simulink model "stateFullOBS"  (Simulink 7.4)
settings: Solver=ode4  StartTime=0.0  StopTime=inf  FixedStep=0.01  RelTol=1e-3
undefined symbols (not defined in the file): A, aarm, apind, B, C, F, Fi, L, M
libraries: xpcnilib x2
settings Model: Creator=Skov  LastModifiedBy=Skov  SimulationMode=external  BufferReuse=off
settings DataIOCC: SaveState=on  InspectSignalLogs=on
settings OptimizationCC: BlockReduction=off  OptimizeBlockIOStorage=off  BufferReuse=off  ExpressionFolding=off  LocalBlockOutputs=off
settings HardwareCC: ProdIntDivRoundTo=Zero  ProdEndianess=LittleEndian  ProdHWDeviceType=Generic->32-bit x86 compatible
settings RTWCC: SystemTargetFile=xpctarget.tlc  TemplateMakefile=xpc_default_tmf  Description=xPC Target  ProcessScript=xpctarget_make_rtw_hook  RTWCompilerOptimization=On
settings xpcTargetCC: TargetFcnLib=ansi_tfl_table_tmw.mat  TargetFunctionLibrary=ANSI_C  ParMdlRefBuildCompliant=off  PortableWordSizes=off  xPCLoadParamSetFile=off

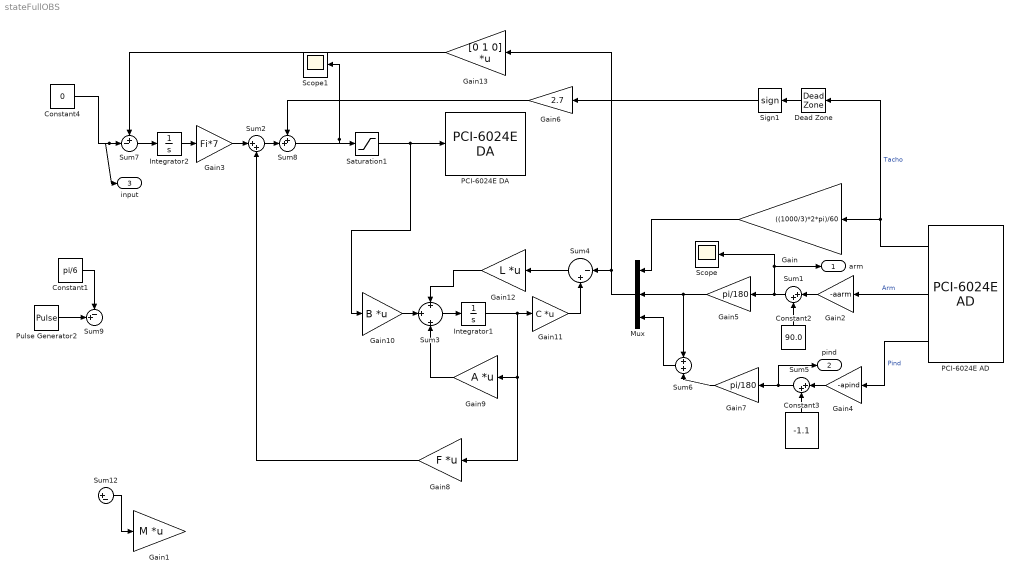
== system stateFullOBS ==
  Constant1 : Constant  Value=pi/6  OutDataType=fixdt(1, 16)  OutScaling=2^0
  Constant2 : Constant  Value=90.0  OutDataType=fixdt(1, 16)  OutScaling=2^0
  Constant3 : Constant  Value=-1.1  OutDataType=fixdt(1, 16)  OutScaling=2^0
  Constant4 : Constant  Value=0  OutDataType=fixdt(1, 16)  OutScaling=2^0
  Dead Zone : DeadZone  LowerValue=-0.01  UpperValue=0.01  SaturateOnIntegerOverflow=on
  Gain : Gain  Gain=((1000/3)*2*pi)/60  ParameterDataType=fixdt(1, 16)  ParameterScaling=2^0  OutDataType=fixdt(1, 16)  OutScaling=2^0
  Gain1 : Gain  Gain=M  Multiplication=Matrix(K*u)  ParameterDataType=fixdt(1, 16)  ParameterScaling=2^0  OutDataType=fixdt(1, 16)  OutScaling=2^0
  Gain10 : Gain  Gain=B  Multiplication=Matrix(K*u)  ParameterDataType=fixdt(1, 16)  ParameterScaling=2^0  OutDataType=fixdt(1, 16)  OutScaling=2^0
  Gain11 : Gain  Gain=C  Multiplication=Matrix(K*u)  ParameterDataType=fixdt(1, 16)  ParameterScaling=2^0  OutDataType=fixdt(1, 16)  OutScaling=2^0
  Gain12 : Gain  Gain=L  Multiplication=Matrix(K*u)  ParameterDataType=fixdt(1, 16)  ParameterScaling=2^0  OutDataType=fixdt(1, 16)  OutScaling=2^0
  Gain13 : Gain  Gain=[0 1 0]  Multiplication=Matrix(K*u)  ParameterDataType=fixdt(1, 16)  ParameterScaling=2^0  OutDataType=fixdt(1, 16)  OutScaling=2^0
  Gain2 : Gain  Gain=-aarm  ParameterDataType=fixdt(1, 16)  ParameterScaling=2^0  OutDataType=fixdt(1, 16)  OutScaling=2^0
  Gain3 : Gain  Gain=Fi*7  ParameterDataType=fixdt(1, 16)  ParameterScaling=2^0  OutDataType=fixdt(1, 16)  OutScaling=2^0
  Gain4 : Gain  Gain=-apind  ParameterDataType=fixdt(1, 16)  ParameterScaling=2^0  OutDataType=fixdt(1, 16)  OutScaling=2^0
  Gain5 : Gain  Gain=pi/180  ParameterDataType=fixdt(1, 16)  ParameterScaling=2^0  OutDataType=fixdt(1, 16)  OutScaling=2^0
  Gain6 : Gain  Gain=2.7  ParameterDataType=fixdt(1, 16)  ParameterScaling=2^0  OutDataType=fixdt(1, 16)  OutScaling=2^0
  Gain7 : Gain  Gain=pi/180  ParameterDataType=fixdt(1, 16)  ParameterScaling=2^0  OutDataType=fixdt(1, 16)  OutScaling=2^0
  Gain8 : Gain  Gain=F  Multiplication=Matrix(K*u)  ParameterDataType=fixdt(1, 16)  ParameterScaling=2^0  OutDataType=fixdt(1, 16)  OutScaling=2^0
  Gain9 : Gain  Gain=A  Multiplication=Matrix(K*u)  ParameterDataType=fixdt(1, 16)  ParameterScaling=2^0  OutDataType=fixdt(1, 16)  OutScaling=2^0
  Integrator1 : Integrator  InitialCondition=[0 0 0 0]
  Integrator2 : Integrator  InitialCondition=[0]
  Mux : Mux  Inputs=3
  PCI-6024E AD : xpcnilib/A//D/E Series/PCI-6024E AD  channel=[3 1 2]  range=[-10]  coupling=[0]  sampletime=0.01  slot=-1
  PCI-6024E DA : xpcnilib/D//A/E Series/PCI-6024E DA  channel=[1]  reset=[1]  initValue=[0]  sampletime=0.01  slot=-1
  Pulse Generator2 : DiscretePulseGenerator  PulseType=Time based  Amplitude=pi/3  Period=40  PulseWidth=50  PhaseDelay=0  SampleTime=1
  Saturation1 : Saturate  UpperLimit=10  LowerLimit=-10  OutDataType=fixdt(1, 16)  OutScaling=2^0
  Scope : Scope
      settings: YMin=-35  YMax=35
  Scope1 : Scope
      settings: YMin=-20  YMax=40
  Sign1 : Signum
  Sum1 : Sum  Inputs=|++  OutDataType=fixdt(1, 16)  OutScaling=2^0
  Sum12 : Sum  Inputs=|+-  OutDataType=fixdt(1, 16)  OutScaling=2^0
  Sum2 : Sum  Inputs=|++  OutDataType=fixdt(1, 16)  OutScaling=2^0
  Sum3 : Sum  Inputs=+|+|+  OutDataType=fixdt(1, 16)  OutScaling=2^0
  Sum4 : Sum  Inputs=|-+  OutDataType=fixdt(1, 16)  OutScaling=2^0
  Sum5 : Sum  Inputs=|++  OutDataType=fixdt(1, 16)  OutScaling=2^0
  Sum6 : Sum  Inputs=+|+  OutDataType=fixdt(1, 16)  OutScaling=2^0
  Sum7 : Sum  Inputs=+-|  OutDataType=fixdt(1, 16)  OutScaling=2^0
  Sum8 : Sum  Inputs=++|  OutDataType=fixdt(1, 16)  OutScaling=2^0
  Sum9 : Sum  Inputs=-+|  OutDataType=fixdt(1, 16)  OutScaling=2^0
  arm : Outport  OutDataType=fixdt(1, 16)  OutScaling=2^0
  pind : Outport  Port=2  OutDataType=fixdt(1, 16)  OutScaling=2^0
  input : Outport  Port=3  OutDataType=fixdt(1, 16)  OutScaling=2^0
  wires:
  Gain2/1 -> Sum1/1
  Constant2/1 -> Sum1/2
  Sum1/1 -> Gain5/1, arm/1, Scope/1
  PCI-6024E AD/1 -> Gain/1, Dead Zone/1  "Tacho"
  PCI-6024E AD/2 -> Gain2/1  "Arm"
  PCI-6024E AD/3 -> Gain4/1  "Pind"
  Gain4/1 -> Sum5/1
  Constant3/1 -> Sum5/2
  Sum5/1 -> Gain7/1, pind/1
  Integrator1/1 -> Gain11/1, Gain8/1, Gain9/1
  Sum3/1 -> Integrator1/1
  Gain9/1 -> Sum3/3
  Gain10/1 -> Sum3/2
  Sum4/1 -> Gain12/1
  Gain11/1 -> Sum4/2
  Gain8/1 -> Sum2/2
  Gain13/1 -> Sum7/1
  Gain5/1 -> Mux/2, Sum6/1
  Gain/1 -> Mux/1
  Mux/1 -> Gain13/1, Sum4/1
  Gain7/1 -> Sum6/2
  Sum6/1 -> Mux/3
  Dead Zone/1 -> Sign1/1
  Sign1/1 -> Gain6/1
  Sum2/1 -> Sum8/2
  Gain6/1 -> Sum8/1
  Sum8/1 -> Scope1/1, Saturation1/1
  Integrator2/1 -> Gain3/1
  Constant4/1 -> Sum7/2, input/1
  Sum7/1 -> Integrator2/1
  Gain3/1 -> Sum2/1
  Saturation1/1 -> PCI-6024E DA/1, Gain10/1
  Gain12/1 -> Sum3/1
  Sum12/1 -> Gain1/1
  Constant1/1 -> Sum9/1
  Pulse Generator2/1 -> Sum9/2
